simulink model "BPSK_RX_Nishat"  (R2018a)
settings: Solver=VariableStepAuto  StartTime=0.0  StopTime=inf  RelTol=1e-3
undefined symbols (not defined in the file): BitRate
libraries: commrfcorlib x2, commsync2 x2, sdrublksprivate x1, commdigbbndpm3 x1, commfilt2 x1, commsdrhw_v2 x1
settings Model: Creator=n53s123  LastModifiedBy=n53s123

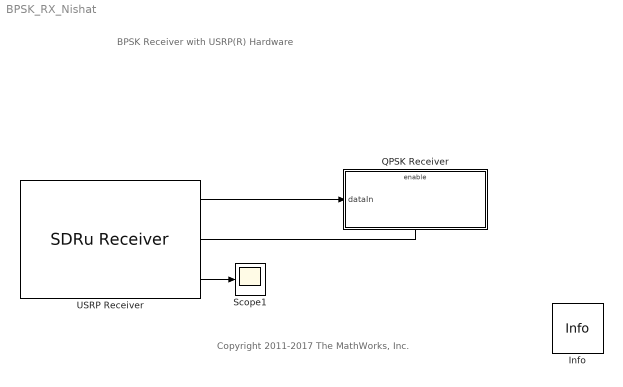
== system BPSK_RX_Nishat ==
  note: BPSK Receiver with USRP(R) Hardware
  note: Copyright 2011-2017 The MathWorks, Inc.
  Info : sdrublksprivate/Info  SystemSampleTime=-1
      settings: SourceProductName=Communications System Toolbox Support Package for USRP(R) Radio  SourceProductBaseCode=USRP
  QPSK Receiver : Subsystem
      mask Display: disp('BPSK Receiver')
  Scope1 : Scope
  USRP Receiver : commsdrhw_v2/SDRu Receiver  SourceLibraryInfo="This block requires <a href=\"http://www.mathworks.com/hardware-support/usrp.html\">Communications System Toolbox Support Package for USRP Radio</a>"  rxtx=rx  initializeIPAddress=0  devMap=0  USRP2_IP=192.168.10.2  USRP_IP_X300=192.168.10.2  USRP_IP_X310=192.168.10.2  USRP_serialNumB200=30B2ACA  USRP_serialNumB210=ECR04ZDBT  platform=N200/N210/USRP2  prevPlatform=N200/N210/USRP2  lastIPAddressPopup=192.168.10.2  USRP_ID=192.168.10.2  LastIPAddress=192.168.10.2  ChannelMapping=1  centerFrequencySrc=Dialog  centerFrequency=15e6  loOffsetSrc=Dialog  loOffset=0  gainSrc=Dialog  gain=0  PPSSource=Internal  clockSource=Internal  masterClkRateParam=100e6  masterClkRateB200=sdrqpskrx.MasterClockRate  masterClkRateB210=sdrqpskrx.MasterClockRate  masterClkRateX300=200e6  masterClkRateX310=200e6  masterClkRate=100e6  decimInterpSrc=Dialog  decimInterp=500  USRP2_IP_NUM=[49 57 50 46 49 54 56 46 49 48 46 50]  TransportDataType=int16  overrunUnderrunPort=on  sampleTime=1/BitRate*4000  outputDatatype=single  frameLength=4000  HOST_DATA_PORT=0  HOST_CONTROL_PORT=0  USRP2_DATA_PORT=0  USRP2_CONTROL_PORT=0  bufferMode=Continuous streaming  EnableBurstMode=off  NumFramesInBurst=100
      settings: SourceProductName=Communications System Toolbox Support Package for USRP(R) Radio  SourceProductBaseCode=USRP
  wires:
  USRP Receiver/3 -> Scope1/1
  USRP Receiver/1 -> QPSK Receiver/1(dataIn)
  USRP Receiver/2 -> QPSK Receiver/Enable

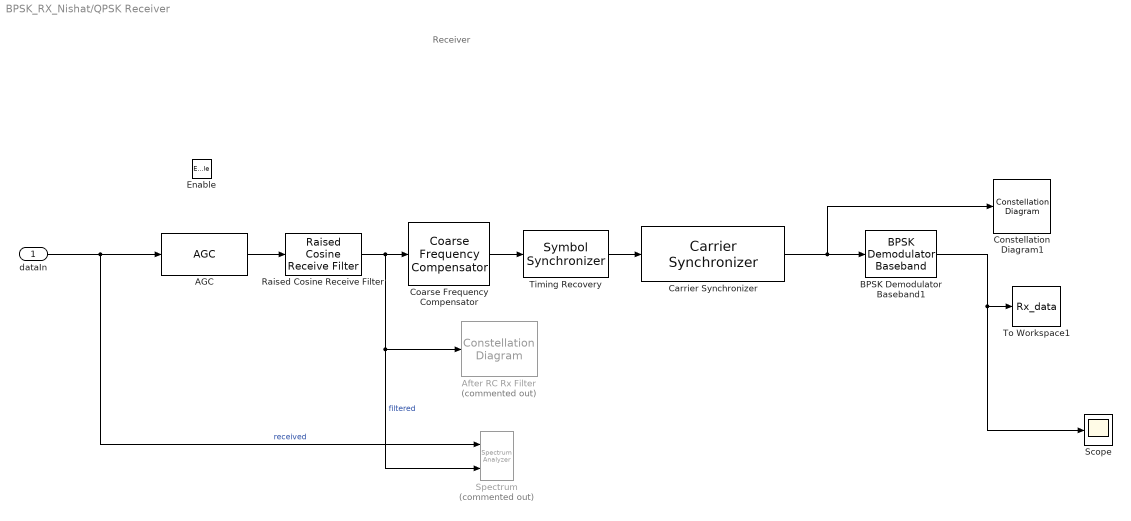
== system BPSK_RX_Nishat/QPSK Receiver ==
  note: Receiver
  dataIn : Inport
  Enable : EnablePort  PropagateVarSize=During execution
  AGC : commrfcorlib/AGC  LegacyMode=off  DetectorMethod=Rectifier  LoopMethod=Linear  UpdatePeriod=100  StepSize=0.1  AdaptationStepSize=0.01  DesiredOutputPower=2  AveragingLength=50  MaximumGain=30  MaxPowerGain=60  GainOutputPort=off  InputPowerOutputPort=off  SimulateUsing=Code generation
      settings: SourceProductName=Communications System Toolbox
  After RC Rx Filter : ConstellationDiagram  Tag=ScatterPlot  Commented=on
  BPSK Demodulator Baseband1 : commdigbbndpm3/BPSK Demodulator Baseband  DecType=Hard decision  VarSource=Dialog  Variance=1  Ph=0  outDtype=Inherit via internal rule  derotateFactorWordLen=16  derotateFactorDataTypeStr=Inherit: Same word length as input  derotateFactorLastDataTypeStr=Inherit: Same word length as input
  Carrier Synchronizer : commsync2/Carrier Synchronizer  Modulation=BPSK  ModulationPhaseOffset=Auto  CustomPhaseOffset=0  SamplesPerSymbol=2  DampingFactor=0.707  NormalizedLoopBandwidth=0.01  EstimatedPhaseErrorOutputPort=off  SimulateUsing=Code generation
      settings: SourceProductName=Communications System Toolbox
  Coarse Frequency Compensator : commrfcorlib/Coarse Frequency Compensator  Modulation=BPSK  Algorithm=FFT-based  FrequencyResolution=0.001  MaximumFrequencyOffset=0.05  SamplesPerSymbol=4  EstimatedFreqOffsetPort=off  SimulateUsing=Code generation
      settings: SourceProductName=Communications System Toolbox  SourceProductBaseCode=CM
  Constellation Diagram1 : ConstellationDiagram
  Raised Cosine Receive Filter : commfilt2/Raised Cosine Receive Filter  filtType=Square root  R=0.5  filtSpan=10  N=2  downFactor=1  downOffset=0  filterGain=1  InputProcessing=Columns as channels (frame based)  RateOptions=Enforce single-rate processing  framing=Mute  checkCoeff=off  variableName=rcRxFilt  currentFiltSpan=10  D=5  inputOffset=0  sampMode=Mute  saveAsFlag=0  rateMode=Downsampling  checkGain=Normalized  launchFVT=on  roundingMode=Floor  overflowMode=off  coeffDataTypeStr=Inherit: Same word length as input  coeffMin=[]  coeffMax=[]  coeffLastDataTypeStr=Inherit: Same word length as input  accumDataTypeStr=Inherit: Same as product output  accumLastDataTypeStr=Inherit: Same as product output  outputDataTypeStr=Inherit: Same as accumulator  outputMin=[]  outputMax=[]  outputLastDataTypeStr=Inherit: Same as accumulator
  Scope : Scope
  Spectrum : SpectrumAnalyzer  Commented=on  NumInputPorts=2
  Timing Recovery : commsync2/Symbol Synchronizer  Modulation=PAM/PSK/QAM  TimingErrorDetector=Gardner (non-data-aided)  SamplesPerSymbol=2  DampingFactor=1  NormalizedLoopBandwidth=0.01  DetectorGain=5.4  TimingErrorOutputPort=off  SimulateUsing=Code generation
      settings: SourceProductName=Communications System Toolbox  SourceProductBaseCode=CM
  To Workspace1 : ToWorkspace  VariableName=Rx_data  SaveFormat=Structure With Time  SampleTime=-1
  wires:
  Raised Cosine Receive Filter/1 -> Coarse Frequency Compensator/1, After RC Rx Filter/1, Spectrum/2  "filtered"
  AGC/1 -> Raised Cosine Receive Filter/1
  Timing Recovery/1 -> Carrier Synchronizer/1
  dataIn/1 -> AGC/1, Spectrum/1  "received"
  Coarse Frequency Compensator/1 -> Timing Recovery/1
  Carrier Synchronizer/1 -> Constellation Diagram1/1, BPSK Demodulator Baseband1/1
  BPSK Demodulator Baseband1/1 -> Scope/1, To Workspace1/1
